simulink library "groundStation000_cl"  (R2018b)
settings: Solver=VariableStepAuto  StartTime=0.0  StopTime=10.0  RelTol=1e-3
libraries: eulAng2RotMat_ul x1, massSpringDamper_ul x1, tethersMoment_cl x1, thrAttachPtKinematics_ul x1
settings Model: Creator=M.Cobb  LastModifiedBy=mcobb

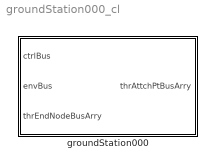
== system groundStation000_cl ==
  groundStation000 : Subsystem  mask{gs=0}
      mask prompts: gs "Ground station object"

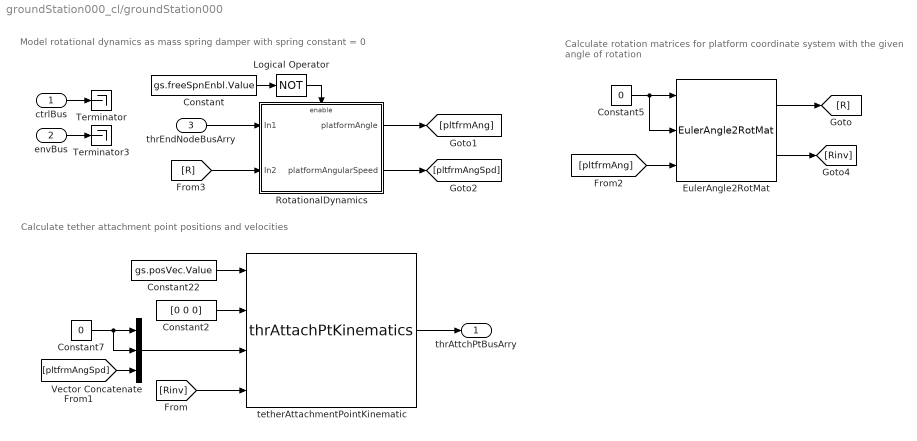
== system groundStation000_cl/groundStation000 ==
  note: Calculate tether attachment point positions and velocities
  note: Calculate rotation matrices for platform coordinate
      | system with the given angle of rotation
  note: Model rotational dynamics as mass spring damper with
      | spring constant = 0
  ctrlBus : Inport  OutDataTypeStr=Bus: ctrlBus
  envBus : Inport  Port=2  OutDataTypeStr=Bus: envBus
  thrEndNodeBusArry : Inport  Port=3
  Constant : Constant  Value=gs.freeSpnEnbl.Value
  Constant2 : Constant  Value=[0 0 0]
  Constant22 : Constant  Value=gs.posVec.Value
  Constant5 : Constant  Value=0
  Constant7 : Constant  Value=0
  EulerAngle2RotMat : eulAng2RotMat_ul/EulerAngle2RotMat  SystemSampleTime=-1
  Logical Operator : Logic  Operator=NOT  AllPortsSameDT=off  OutDataTypeStr=boolean
  RotationalDynamics : Subsystem
      settings: MinAlgLoopOccurrences=on
  Terminator : Terminator
  Terminator3 : Terminator
  Vector Concatenate : Concatenate  NumInputs=3
  tetherAttachmentPointKinematic : thrAttachPtKinematics_ul/thrAttachPtKinematics  atchPts=gs.struct('groundStation.thrAttach')
  thrAttchPtBusArry : Outport
  wires:
  Constant5/1 -> EulerAngle2RotMat/2, EulerAngle2RotMat/1
  EulerAngle2RotMat/1 -> [R]
  EulerAngle2RotMat/2 -> [Rinv]
  Constant7/1 -> Vector Concatenate/1, Vector Concatenate/2
  tetherAttachmentPointKinematic/1 -> thrAttchPtBusArry/1
  Constant22/1 -> tetherAttachmentPointKinematic/1
  Constant2/1 -> tetherAttachmentPointKinematic/2
  [Rinv] -> tetherAttachmentPointKinematic/4
  Vector Concatenate/1 -> tetherAttachmentPointKinematic/3
  [pltfrmAngSpd] -> Vector Concatenate/3
  [pltfrmAng] -> EulerAngle2RotMat/3
  ctrlBus/1 -> Terminator/1
  envBus/1 -> Terminator3/1
  Constant/1 -> Logical Operator/1
  Logical Operator/1 -> RotationalDynamics/Enable
  thrEndNodeBusArry/1 -> RotationalDynamics/1(In1)
  [R] -> RotationalDynamics/2(In2)
  RotationalDynamics/1(platformAngle) -> [pltfrmAng]
  RotationalDynamics/2(platformAngularSpeed) -> [pltfrmAngSpd]

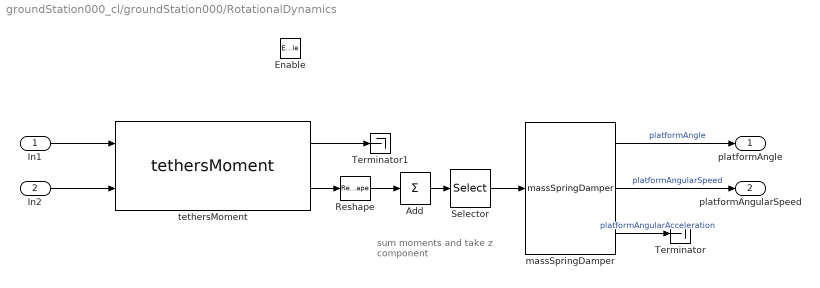
== system groundStation000_cl/groundStation000/RotationalDynamics ==
  note: sum moments and
      | take z component
  In1 : Inport
  In2 : Inport  Port=2
  Enable : EnablePort
  Add : Sum  Inputs=+  CollapseMode=Specified dimension  CollapseDim=2
  Reshape : Reshape  OutputDimensionality=Customize  OutputDimensions=[3 gs.numTethers.Value]
  Selector : Selector  InputPortWidth=3  IndexOptions=Index vector (dialog)  Indices=3  OutputSizes=1
  Terminator : Terminator
  Terminator1 : Terminator
  massSpringDamper : massSpringDamper_ul/massSpringDamper  m=gs.inertia.Value  b=gs.dampCoeff.Value  k=0  x0=gndStn.initAngPos.Value  xDot0=gndStn.initAngPos.Value
  tethersMoment : tethersMoment_cl/tethersMoment  arms=gs.struct('groundStation.thrAttach')
  platformAngle : Outport  InitialOutput=gs.initAngPos.Value
  platformAngularSpeed : Outport  Port=2  InitialOutput=gs.initAngVel.Value
  wires:
  massSpringDamper/2 -> platformAngularSpeed/1  "platformAngularSpeed"
  Add/1 -> Selector/1
  Selector/1 -> massSpringDamper/1
  Reshape/1 -> Add/1
  tethersMoment/1 -> Terminator1/1
  tethersMoment/2 -> Reshape/1
  In1/1 -> tethersMoment/1
  In2/1 -> tethersMoment/2
  massSpringDamper/1 -> platformAngle/1  "platformAngle"
  massSpringDamper/3 -> Terminator/1  "platformAngularAcceleration"
